simulink model "two_virtual_wheel_discrete"  (R2020a)
settings: Solver=ode3  StartTime=0.0  StopTime=tfinal  FixedStep=.002  RelTol=1e-3  EnableMultiTasking=on
values from neighbouring files (symbols this model uses):
  b1 = T1*k1    (= 0.15)    [two_virtual_wheel_params.m]
  b2 = T2*k2    (= 0.0075)    [two_virtual_wheel_params.m]
  Jw1 = .5*1.5/4    (= 0.1875)    [two_virtual_wheel_params.m]
  Jw2 = 0.0721    [two_virtual_wheel_params.m]
  k1 = .5*15    (= 7.5)    [two_virtual_wheel_params.m]
  k2 = 3.75    [two_virtual_wheel_params.m]
  step_time = 1    [two_virtual_wheel_params.m]
  T1 = 1/50    (= 0.02)    [two_virtual_wheel_params.m]
  T2 = 1/500    (= 0.002)    [two_virtual_wheel_params.m]
  Theta_z_0 = 45    [two_virtual_wheel_params.m]
undefined symbols (not defined in the file or in its folder): DiscIntNeverNeededParam
settings Model: ExtModeTrigMode=oneshot  ExtModeArmWhenConnect=off  Creator=jfr  LastModifiedBy=ecs
settings DataIOCC: SaveFormat=Array  SignalLoggingSaveFormat=ModelDataLogs  ReturnWorkspaceOutputs=off  SignalLoggingName=sigsOut
settings OptimizationCC: BooleanDataType=off  ExpressionDepthLimit=2147483647  InitFltsAndDblsToZero=on  LifeSpan=inf
settings DebuggingCC: SaveWithParameterizedLinksMsg=none  UnderspecifiedInitializationDetection=Classic  MergeDetectMultiDrivingBlocksExec=none  SignalResolutionControl=TryResolveAllWithWarning  MultiTaskDSMMsg=warning  MultiTaskCondExecSysMsg=none  FcnCallInpInsideContextMsg=warning  AllowSymbolicDim=off  StateNameClashWarn=warning  SFUnexpectedBacktrackingDiag=warning  SFNoUnconditionalDefaultTransitionDiag=warning  SFExecutionAtInitializationDiag=none  ArithmeticOperatorsInVariantConditions=warning
settings HardwareCC: ProdBitPerPointer=32  ProdBitPerSizeT=32  ProdBitPerPtrDiffT=32  ProdLargestAtomicFloat=None  ProdIntDivRoundTo=Undefined  ProdEndianess=Unspecified  ProdWordSize=32  ProdHWDeviceType=32-bit Generic  TargetUnknown=on
settings ModelReferenceCC: PropagateSignalLabelsOutOfModel=off
settings SFSimCC: SimUseLocalCustomCode=off  CustomCodeUndefinedFunction=UseInterfaceOnly
settings RTWCC: RTWUseLocalCustomCode=off
settings CodeAppCC: StateflowObjectComments=on
settings GRTTargetCC: TargetFcnLib=ansi_tfl_tmw.mat  TargetLangStandard=C89/C90 (ANSI)  CombineOutputUpdateFcns=off  GRTInterface=on
settings ConfigComp: CovMetricSettings=dw  CovHtmlReporting=on  CovSaveCumulativeToWorkspaceVar=on  CovSaveSingleToWorkspaceVar=on  CovExternalEMLEnable=off

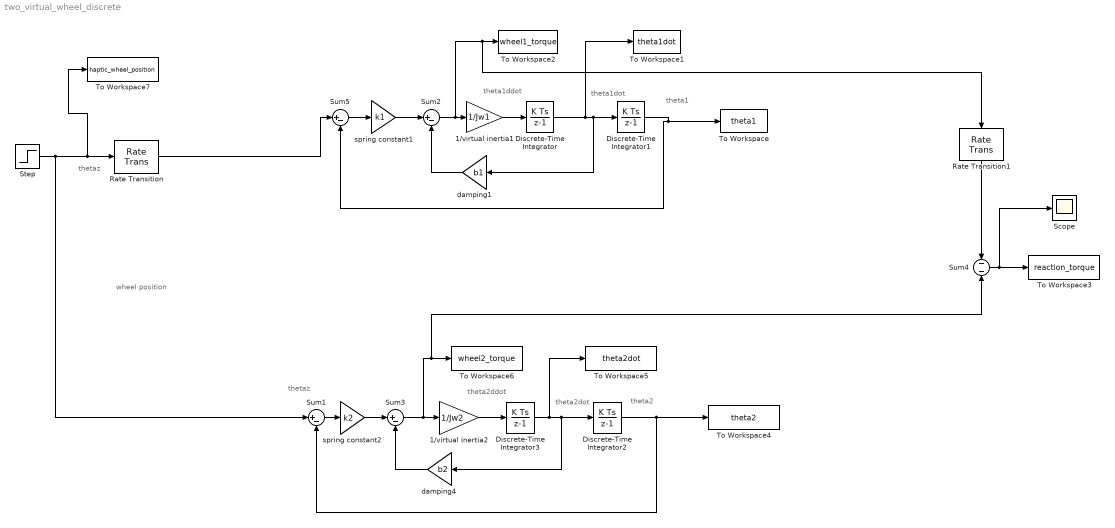
== system two_virtual_wheel_discrete ==
  note: thetaz
  note: wheel position
  note: thetaz
  note: theta2ddot
  note: theta2dot
  note: theta2
  note: theta1dot
  note: theta1ddot
  note: theta1
  1/virtual inertia1 : Gain  Gain=1/Jw1  SaturateOnIntegerOverflow=on  OutDataTypeStr=Inherit: Same as input  ParamDataTypeStr=Inherit: Same as input
  1/virtual inertia2 : Gain  Gain=1/Jw2  SaturateOnIntegerOverflow=on  OutDataTypeStr=Inherit: Same as input  ParamDataTypeStr=Inherit: Same as input
  Discrete-Time Integrator : DiscreteIntegrator  SampleTime=T1  ICPrevOutput=DiscIntNeverNeededParam  ICPrevScaledInput=DiscIntNeverNeededParam
  Discrete-Time Integrator1 : DiscreteIntegrator  SampleTime=T1  ICPrevOutput=DiscIntNeverNeededParam  ICPrevScaledInput=DiscIntNeverNeededParam
  Discrete-Time Integrator2 : DiscreteIntegrator  SampleTime=T2  ICPrevOutput=DiscIntNeverNeededParam  ICPrevScaledInput=DiscIntNeverNeededParam
  Discrete-Time Integrator3 : DiscreteIntegrator  SampleTime=T2  ICPrevOutput=DiscIntNeverNeededParam  ICPrevScaledInput=DiscIntNeverNeededParam
  Rate Transition : RateTransition
  Rate Transition1 : RateTransition
  Scope : Scope
  Step : Step  Time=step_time  After=Theta_z_0  SampleTime=T2
  Sum{1..3,5} (4 alike) : Sum  Inputs=|+-  InputSameDT=on  SaturateOnIntegerOverflow=on  OutDataTypeStr=Inherit: Same as first input
  Sum4 : Sum  Inputs=-|-  InputSameDT=on  SaturateOnIntegerOverflow=on  OutDataTypeStr=Inherit: Same as first input
  To Workspace : ToWorkspace  VariableName=theta1  SaveFormat=Timeseries  SampleTime=-1
  To Workspace1 : ToWorkspace  VariableName=theta1dot  SaveFormat=Timeseries  SampleTime=-1
  To Workspace2 : ToWorkspace  VariableName=wheel1_torque  SaveFormat=Timeseries  SampleTime=-1
  To Workspace3 : ToWorkspace  VariableName=reaction_torque  SaveFormat=Timeseries  SampleTime=-1
  To Workspace4 : ToWorkspace  VariableName=theta2  SaveFormat=Timeseries  SampleTime=-1
  To Workspace5 : ToWorkspace  VariableName=theta2dot  SaveFormat=Timeseries  SampleTime=-1
  To Workspace6 : ToWorkspace  VariableName=wheel2_torque  SaveFormat=Timeseries  SampleTime=-1
  To Workspace7 : ToWorkspace  VariableName=haptic_wheel_position  SaveFormat=Timeseries  SampleTime=-1
  damping1 : Gain  Gain=b1  SaturateOnIntegerOverflow=on  OutDataTypeStr=Inherit: Same as input  ParamDataTypeStr=Inherit: Same as input
  damping4 : Gain  Gain=b2  SaturateOnIntegerOverflow=on  OutDataTypeStr=Inherit: Same as input  ParamDataTypeStr=Inherit: Same as input
  spring constant1 : Gain  Gain=k1  SaturateOnIntegerOverflow=on  OutDataTypeStr=Inherit: Same as input  ParamDataTypeStr=Inherit: Same as input
  spring constant2 : Gain  Gain=k2  SaturateOnIntegerOverflow=on  OutDataTypeStr=Inherit: Same as input  ParamDataTypeStr=Inherit: Same as input
  wires:
  Sum4/1 -> Scope/1, To Workspace3/1
  Rate Transition1/1 -> Sum4/1
  spring constant2/1 -> Sum3/1
  Sum1/1 -> spring constant2/1
  damping4/1 -> Sum3/2
  Discrete-Time Integrator3/1 -> To Workspace5/1, Discrete-Time Integrator2/1, damping4/1
  Step/1 -> Sum1/1, To Workspace7/1, Rate Transition/1
  1/virtual inertia2/1 -> Discrete-Time Integrator3/1
  Discrete-Time Integrator2/1 -> To Workspace4/1, Sum1/2
  Sum3/1 -> 1/virtual inertia2/1, Sum4/2, To Workspace6/1
  Rate Transition/1 -> Sum5/1
  Discrete-Time Integrator1/1 -> Sum5/2, To Workspace/1
  spring constant1/1 -> Sum2/1
  Sum2/1 -> 1/virtual inertia1/1, Rate Transition1/1, To Workspace2/1
  Sum5/1 -> spring constant1/1
  1/virtual inertia1/1 -> Discrete-Time Integrator/1
  damping1/1 -> Sum2/2
  Discrete-Time Integrator/1 -> Discrete-Time Integrator1/1, damping1/1, To Workspace1/1
